simulink model "control_simulation"  (R2016a)
settings: Solver=ode4  StartTime=0.0  StopTime=Tfinal  FixedStep=Ts  RelTol=1e-3
values from neighbouring files (symbols this model uses):
  Cdc = 100e-6    (= 0.0001)    [control_simulation_parameters.m]    (also in pmsm_vbyf_sim_parameters.m = 1.5e-05; vbyfcontrolim_sim.m)
  delta = acos(Ef/Vt)    [control_simulation_parameters.m]    (also in pmsm_vbyf_sim_parameters.m; vbyfcontrolim_sim.m = 0)
  deltad = delta*180/pi    [control_simulation_parameters.m]    (also in pmsm_vbyf_sim_parameters.m)
  Ef = 155    [control_simulation_parameters.m]    (also in pmsm_vbyf_sim_parameters.m = 80)
  fout = 100    [control_simulation_parameters.m]    (also in pmsm_vbyf_sim_parameters.m; vbyfcontrolim_sim.m = 50)
  fsw = 10e3    (= 10000)    [control_simulation_parameters.m]    (also in pmsm_vbyf_sim_parameters.m; vbyfcontrolim_sim.m)
  Ls = 13.8e-3    (= 0.0138)    [control_simulation_parameters.m]
  ma = Vt*sqrt(3)/(Vdcm*0.612)    [control_simulation_parameters.m]    (also in pmsm_vbyf_sim_parameters.m; vbyfcontrolim_sim.m = 0.9)
  motor_speed = 600    [control_simulation_parameters.m]
  phase = [0 90 0 90]    [control_simulation_parameters.m]    (also in pmsm_vbyf_sim_parameters.m = [0])
  Rin = 10    [control_simulation_parameters.m]    (also in pmsm_vbyf_sim_parameters.m = 1; vbyfcontrolim_sim.m = 1e-06)
  Ripth = 0.08    [control_simulation_parameters.m]    (also in pmsm_vbyf_sim_parameters.m; vbyfcontrolim_sim.m)
  Rs = 1e-3    (= 0.001)    [control_simulation_parameters.m]
  Ts = 1e-6    (= 1e-06)    [control_simulation_parameters.m]    (also in pmsm_vbyf_sim_parameters.m; vbyfcontrolim_sim.m)
  Vin = Vdc + Rin*(Pout/Vdc)    (= 697.604412924)    [control_simulation_parameters.m]    (also in pmsm_vbyf_sim_parameters.m = 276.981317008; vbyfcontrolim_sim.m = 750)
  wout = 2*pi*fout    (= 628.318530718)    [control_simulation_parameters.m]    (also in pmsm_vbyf_sim_parameters.m; vbyfcontrolim_sim.m = 314.159265359)
undefined symbols (not defined in the file or in its folder): Lload, Rload
libraries: powerlib x24, powerlib_meascontrol x19, simulink x2
settings Model: Creator=ugurm  LastModifiedBy=mesutto
settings DataIOCC: LimitDataPoints=on  SaveFormat=Array
settings DebuggingCC: UnderspecifiedInitializationDetection=Classic  MergeDetectMultiDrivingBlocksExec=none  SolverPrmCheckMsg=warning  StateNameClashWarn=warning
settings HardwareCC: ProdBitPerPointer=32  ProdLargestAtomicFloat=None  ProdIntDivRoundTo=Undefined  ProdEndianess=Unspecified  ProdWordSize=32  ProdHWDeviceType=32-bit Generic
settings ModelReferenceCC: PropagateSignalLabelsOutOfModel=off
settings ConfigComp: CovModelRefEnable=Off

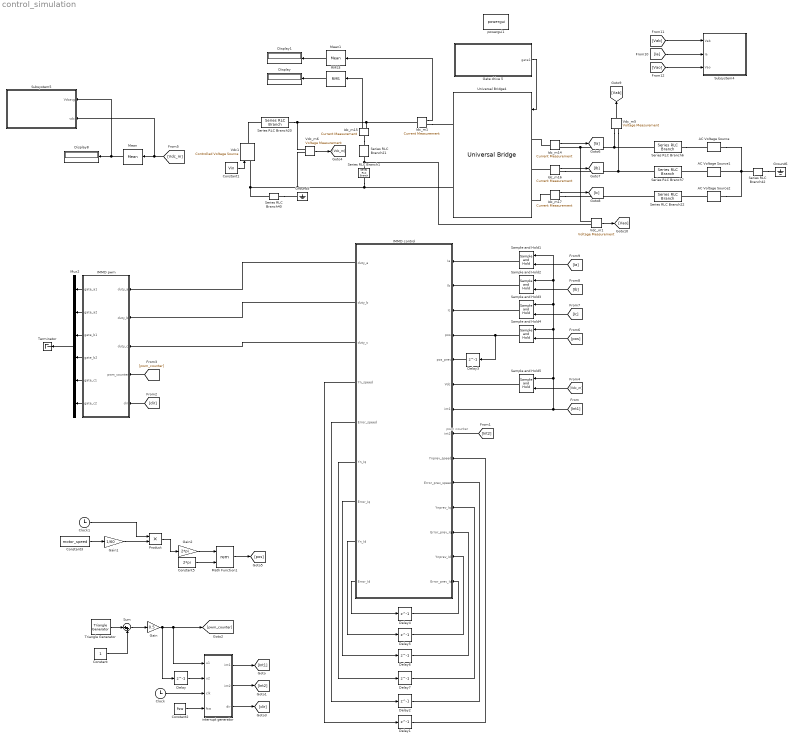
== system control_simulation ==
  note: pwm counter
  AC Voltage Source : powerlib/Electrical Sources/AC Voltage Source  Amplitude=Ef*sqrt(2)  Phase=0  Frequency=fout  SampleTime=0  Measurements=None  BusType=swing  Pref=10e3  Qref=0  Qmin=-inf  Qmax=+inf
  AC Voltage Source1 : powerlib/Electrical Sources/AC Voltage Source  Amplitude=Ef*sqrt(2)  Phase=-120  Frequency=fout  SampleTime=0  Measurements=None  BusType=swing  Pref=10e3  Qref=0  Qmin=-inf  Qmax=+inf
  AC Voltage Source2 : powerlib/Electrical Sources/AC Voltage Source  Amplitude=Ef*sqrt(2)  Phase=-240  Frequency=fout  SampleTime=0  Measurements=None  BusType=swing  Pref=10e3  Qref=0  Qmin=-inf  Qmax=+inf
  Clock : Clock
  Clock1 : Clock
  Constant : Constant
  Constant1 : Constant  Value=Vin
  Constant2 : Constant  Value=fsw
  Constant3 : Constant  Value=motor_speed
  Constant5 : Constant  Value=2*pi
  Delay{,1..7} (8 alike) : Delay  DelayLength=1
  Display : Display
  Display1 : Display
  Display8 : Display
  Gain : Gain  Gain=0.5
  Gain1 : Gain  Gain=1/60
  Gain2 : Gain  Gain=2*pi
  Gate drive 5 : Subsystem
  Ground5 : powerlib/Elements/Ground  LConnTagsString=a
  Ground6 : powerlib/Elements/Ground  LConnTagsString=a
  IMMD control : MATLAB Function  TreatAsAtomicUnit=on
  IMMD pwm : MATLAB Function  TreatAsAtomicUnit=on
  Idc_m{1,14..17} (5 alike) : powerlib/Measurements/Current Measurement  PhasorSimulation=off  OutputType=Complex  PSBequivalent=0
  Math Function1 : Math  Operator=rem  SaturateOnIntegerOverflow=on
  Mean : powerlib_meascontrol/Measurements/Mean  Freq=fout  Vinit=0  Ts=0
  Mean1 : powerlib_meascontrol/Measurements/Mean  Freq=fout  Vinit=0  Ts=0
  Mux2 : Mux  Inputs=6
  Product : Product
  RMS3 : powerlib_meascontrol/Measurements/RMS  TrueRMS=on  Freq=fout  RMSInit=0  Ts=0
  Sample and Hold{1..5} (5 alike) : powerlib_meascontrol/Additional Components/Sample and Hold  ic=0  Ts=0
  Series RLC Branch1 : powerlib/Elements/Series RLC Branch  LConnTagsString=__new0  RConnTagsString=__new0  BranchType=C  Resistance=Rload  Inductance=Lload  SetiL0=off  InitialCurrent=0  Capacitance=Cdc*2  Setx0=off  InitialVoltage=0  Measurements=None
  Series RLC Branch20 : powerlib/Elements/Series RLC Branch  LConnTagsString=__new0  RConnTagsString=__new0  BranchType=R  Resistance=Rin  Inductance=Lload  SetiL0=off  InitialCurrent=0  Capacitance=1e-6  Setx0=off  InitialVoltage=0  Measurements=None
  Series RLC Branch21 : powerlib/Elements/Series RLC Branch  LConnTagsString=__new0  RConnTagsString=__new0  BranchType=C  Resistance=Rload  Inductance=Lload  SetiL0=off  InitialCurrent=0  Capacitance=Cdc*2  Setx0=off  InitialVoltage=0  Measurements=None
  Series RLC Branch22 : powerlib/Elements/Series RLC Branch  LConnTagsString=__new0  RConnTagsString=__new0  BranchType=RL  Resistance=Rs  Inductance=Ls  SetiL0=off  InitialCurrent=0  Capacitance=1e-6  Setx0=off  InitialVoltage=0  Measurements=None
  Series RLC Branch40 : powerlib/Elements/Series RLC Branch  LConnTagsString=__new0  RConnTagsString=__new0  BranchType=R  Resistance=1e12  Inductance=Lload  SetiL0=off  InitialCurrent=0  Capacitance=1e-6  Setx0=off  InitialVoltage=0  Measurements=None
  Series RLC Branch42 : powerlib/Elements/Series RLC Branch  LConnTagsString=__new0  RConnTagsString=__new0  BranchType=R  Resistance=1e12  Inductance=Lload  SetiL0=off  InitialCurrent=0  Capacitance=1e-6  Setx0=off  InitialVoltage=0  Measurements=None
  Series RLC Branch6 : powerlib/Elements/Series RLC Branch  LConnTagsString=__new0  RConnTagsString=__new0  BranchType=RL  Resistance=Rs  Inductance=Ls  SetiL0=off  InitialCurrent=0  Capacitance=1e-6  Setx0=off  InitialVoltage=0  Measurements=None
  Series RLC Branch7 : powerlib/Elements/Series RLC Branch  LConnTagsString=__new0  RConnTagsString=__new0  BranchType=RL  Resistance=Rs  Inductance=Ls  SetiL0=off  InitialCurrent=0  Capacitance=1e-6  Setx0=off  InitialVoltage=0  Measurements=None
  Subsystem4 : Subsystem
  Subsystem5 : Subsystem
  Sum : Sum  Inputs=|++
  Terminator : Terminator
  Triangle Generator : powerlib_meascontrol/Pulse & Signal Generators/Triangle Generator  Freq=fsw  Phase=0  Ts=0
  Universal Bridge4 : powerlib/Power Electronics/Universal Bridge  Arms=3  SnubberResistance=1e5  SnubberCapacitance=inf  Device=IGBT / Diodes  Ron=1e-6  Lon=0  ForwardVoltages="[  0  0  ]"  ForwardVoltage=0  GTOparameters=[ 10e-6 , 20e-6 ]  IGBTparameters=[0,0]  Measurements=None  Measurements_2=None  converterType=Rectifier
  Vdc1 : powerlib/Electrical Sources/Controlled Voltage Source  Initialize=off  Source_Type=DC  Amplitude=200  Phase=0  Frequency=0  Measurements=None
  Vdc_m1 : powerlib/Measurements/Voltage Measurement  PhasorSimulation=off  OutputType=Complex  PSBequivalent=0
  Vdc_m5 : powerlib/Measurements/Voltage Measurement  PhasorSimulation=off  OutputType=Complex  PSBequivalent=0
  Vdc_m6 : powerlib/Measurements/Voltage Measurement  PhasorSimulation=off  OutputType=Complex  PSBequivalent=0
  interrupt generator : MATLAB Function  TreatAsAtomicUnit=on
  powergui1 : powerlib/powergui  Priority=1  SimulationMode=Discrete  SolverType=Tustin  SampleTime=Ts  frequency=60  SPID=off  DisableSnubberDevices=off  DisableRonSwitches=off  DisableVfSwitches=off  SwTol=0  DisplayEquations=off  Interpol=off  ExternalGateDelay=off  methode=off  Ts=0  FunctionMessages=off  echomessages=off  HookPort=off  EnableUseOfTLC=off  x0status=blocks  frequencyindice=0  Pbase=100e6  ErrMax=1e-4  Iterations=50  UnitsV=kV  UnitsW=MW  buscounter=0  RestoreLinks=warning  ResistiveCurrentMeasurement=off  Frange=[0:2:500]  Ylog=off  Xlog=on  ShowGrid=off  save=off  variable=ZData  structure=Vdc  ZoomFFT=off  StartTime=0.04  cycles=5  DisplayStyle=5  fundamental=50  FreqAxis=off  MaxFrequency=30000  frequencyindicesteady=1  RmsSteady=1  display=off
  wires:
  Gate drive 5/1(gate1) -> Universal Bridge4/1
  Constant1/1 -> Vdc1/1
  Idc_m15/1 -> RMS3/1
  Vdc_m6/1 -> [Vdc_m]
  RMS3/1 -> Display/1
  Mean/1 -> Subsystem5/1(Vdcavg), Display8/1
  Idc_m1/1 -> Mean1/1
  Mean1/1 -> Display1/1
  Triangle Generator/1 -> Sum/1
  Constant/1 -> Sum/2
  Sum/1 -> Gain/1
  Gain/1 -> [pwm_counter], interrupt generator/1(u1), Delay/1
  Delay/1 -> interrupt generator/2(u2)
  Clock/1 -> interrupt generator/3(clk)
  Constant2/1 -> interrupt generator/4(fsw)
  Idc_m14/1 -> [Ia]
  [Int1] -> IMMD control/7(int1), Sample and Hold4/2, Sample and Hold3/2, Sample and Hold2/2, Sample and Hold1/2, Sample and Hold5/2
  Constant3/1 -> Gain1/1
  Gain1/1 -> Product/2
  Clock1/1 -> Product/1
  Product/1 -> Gain2/1
  Gain2/1 -> Math Function1/1
  Constant5/1 -> Math Function1/2
  IMMD pwm/1(gate_a1) -> Mux2/1
  IMMD pwm/2(gate_a2) -> Mux2/2
  IMMD pwm/3(gate_b1) -> Mux2/3
  IMMD pwm/4(gate_b2) -> Mux2/4
  IMMD pwm/5(gate_c1) -> Mux2/5
  IMMD pwm/6(gate_c2) -> Mux2/6
  Sample and Hold4/1 -> Delay3/1, IMMD control/4(pos)
  Sample and Hold3/1 -> IMMD control/3(Ic)
  Sample and Hold2/1 -> IMMD control/2(Ib)
  Sample and Hold1/1 -> IMMD control/1(Ia)
  Sample and Hold5/1 -> IMMD control/6(Vdc)
  IMMD control/4(Yn_speed) -> Delay1/1
  Delay1/1 -> IMMD control/9(Ynprev_speed)
  IMMD control/5(Error_speed) -> Delay2/1
  Delay2/1 -> IMMD control/10(Error_prev_speed)
  interrupt generator/1(int1) -> [Int1]
  Mux2/1 -> Terminator/1
  Delay3/1 -> IMMD control/5(pos_prev)
  interrupt generator/2(int2) -> [Int2]
  [Int2] -> IMMD control/8(int2)
  [dir] -> IMMD pwm/5(dir)
  interrupt generator/3(dir) -> [dir]
  [pwm_counter] -> IMMD pwm/4(pwm_counter)
  [Vdc_m] -> Sample and Hold5/1
  IMMD control/9(Error_Id) -> Delay4/1
  Delay4/1 -> IMMD control/14(Error_prev_Id)
  Delay5/1 -> IMMD control/13(Ynprev_Id)
  Delay6/1 -> IMMD control/12(Error_prev_Iq)
  Delay7/1 -> IMMD control/11(Ynprev_Iq)
  IMMD control/6(Yn_Iq) -> Delay7/1
  IMMD control/8(Yn_Id) -> Delay5/1
  IMMD control/7(Error_Iq) -> Delay6/1
  IMMD control/3(duty_c) -> IMMD pwm/3(duty_c)
  IMMD control/2(duty_b) -> IMMD pwm/2(duty_b)
  IMMD control/1(duty_a) -> IMMD pwm/1(duty_a)
  [Vdc_m] -> Subsystem5/2(vdc), Mean/1
  [pos] -> Sample and Hold4/1
  Math Function1/1 -> [pos]
  [Ia] -> Sample and Hold1/1
  [Ib] -> Sample and Hold2/1
  [Ic] -> Sample and Hold3/1
  [Ia] -> Subsystem4/2(Ia)
  Idc_m16/1 -> [Ib]
  Idc_m17/1 -> [Ic]
  [Vab] -> Subsystem4/1(Vab)
  [Vao] -> Subsystem4/3(Vao)
  Vdc_m5/1 -> [Vab]
  Vdc_m1/1 -> [Vao]
  connections:
  Vdc_m5/LConn1 -- Idc_m14/RConn1 -- Vdc_m1/LConn1 -- Series RLC Branch6/LConn1
  Universal Bridge4/RConn2 -- Vdc_m6/LConn2 -- Vdc1/LConn1 -- Series RLC Branch40/LConn1 -- Series RLC Branch1/RConn1
  Series RLC Branch42/RConn1 -- Ground6/LConn1
  Series RLC Branch40/RConn1 -- Ground5/LConn1
  Idc_m14/LConn1 -- Universal Bridge4/LConn1
  Idc_m15/LConn1 -- Series RLC Branch21/LConn1
  Vdc1/RConn1 -- Series RLC Branch20/LConn1
  Series RLC Branch6/RConn1 -- AC Voltage Source/RConn1
  AC Voltage Source1/RConn1 -- Series RLC Branch7/RConn1
  AC Voltage Source2/RConn1 -- Series RLC Branch22/RConn1
  Series RLC Branch42/LConn1 -- AC Voltage Source/LConn1 -- AC Voltage Source2/LConn1 -- AC Voltage Source1/LConn1
  Idc_m16/LConn1 -- Universal Bridge4/LConn2
  Idc_m17/LConn1 -- Universal Bridge4/LConn3
  Idc_m17/RConn1 -- Series RLC Branch22/LConn1
  Idc_m16/RConn1 -- Vdc_m5/LConn2 -- Series RLC Branch7/LConn1
  Idc_m1/RConn1 -- Universal Bridge4/RConn1
  Idc_m1/LConn1 -- Series RLC Branch20/RConn1 -- Vdc_m6/LConn1 -- Idc_m15/RConn1
  Series RLC Branch1/LConn1 -- Vdc_m1/LConn2 -- Series RLC Branch21/RConn1

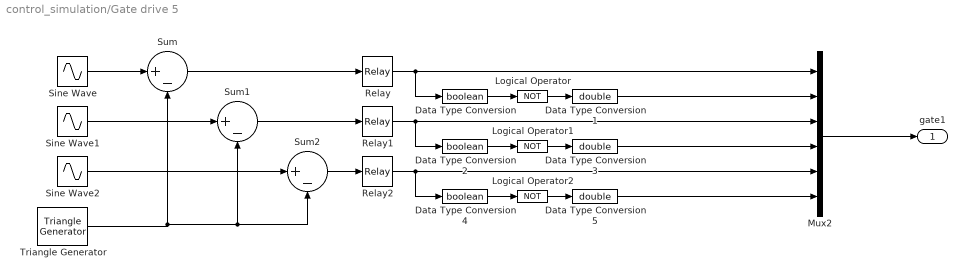
== system control_simulation/Gate drive 5 ==
  Data Type Conversion : DataTypeConversion  OutDataTypeStr=boolean
  Data Type Conversion1 : DataTypeConversion  OutDataTypeStr=double
  Data Type Conversion2 : DataTypeConversion  OutDataTypeStr=boolean
  Data Type Conversion3 : DataTypeConversion  OutDataTypeStr=double
  Data Type Conversion4 : DataTypeConversion  OutDataTypeStr=boolean
  Data Type Conversion5 : DataTypeConversion  OutDataTypeStr=double
  Logical Operator : Logic  Operator=NOT  AllPortsSameDT=off  OutDataTypeStr=boolean
  Logical Operator1 : Logic  Operator=NOT  AllPortsSameDT=off  OutDataTypeStr=boolean
  Logical Operator2 : Logic  Operator=NOT  AllPortsSameDT=off  OutDataTypeStr=boolean
  Mux2 : Mux  Inputs=6
  Relay : Relay
  Relay1 : Relay
  Relay2 : Relay
  Sine Wave : Sin  Amplitude=ma  Frequency=wout  Phase=delta  SampleTime=0
  Sine Wave1 : Sin  Amplitude=ma  Frequency=wout  Phase=-2*pi/3+delta  SampleTime=0
  Sine Wave2 : Sin  Amplitude=ma  Frequency=wout  Phase=2*pi/3+delta  SampleTime=0
  Sum : Sum  Inputs=|+-
  Sum1 : Sum  Inputs=|+-
  Sum2 : Sum  Inputs=|+-
  Triangle Generator : powerlib_meascontrol/Pulse & Signal Generators/Triangle Generator  Freq=fsw  Phase=phase(1)  Ts=Ts
  gate1 : Outport
  wires:
  Sine Wave/1 -> Sum/1
  Triangle Generator/1 -> Sum1/2, Sum2/2, Sum/2
  Sine Wave1/1 -> Sum1/1
  Sine Wave2/1 -> Sum2/1
  Sum/1 -> Relay/1
  Sum1/1 -> Relay1/1
  Sum2/1 -> Relay2/1
  Data Type Conversion/1 -> Logical Operator/1
  Relay/1 -> Data Type Conversion/1, Mux2/1
  Logical Operator/1 -> Data Type Conversion1/1
  Data Type Conversion1/1 -> Mux2/2
  Data Type Conversion2/1 -> Logical Operator1/1
  Relay1/1 -> Data Type Conversion2/1, Mux2/3
  Logical Operator1/1 -> Data Type Conversion3/1
  Data Type Conversion3/1 -> Mux2/4
  Data Type Conversion4/1 -> Logical Operator2/1
  Relay2/1 -> Data Type Conversion4/1, Mux2/5
  Logical Operator2/1 -> Data Type Conversion5/1
  Data Type Conversion5/1 -> Mux2/6
  Mux2/1 -> gate1/1

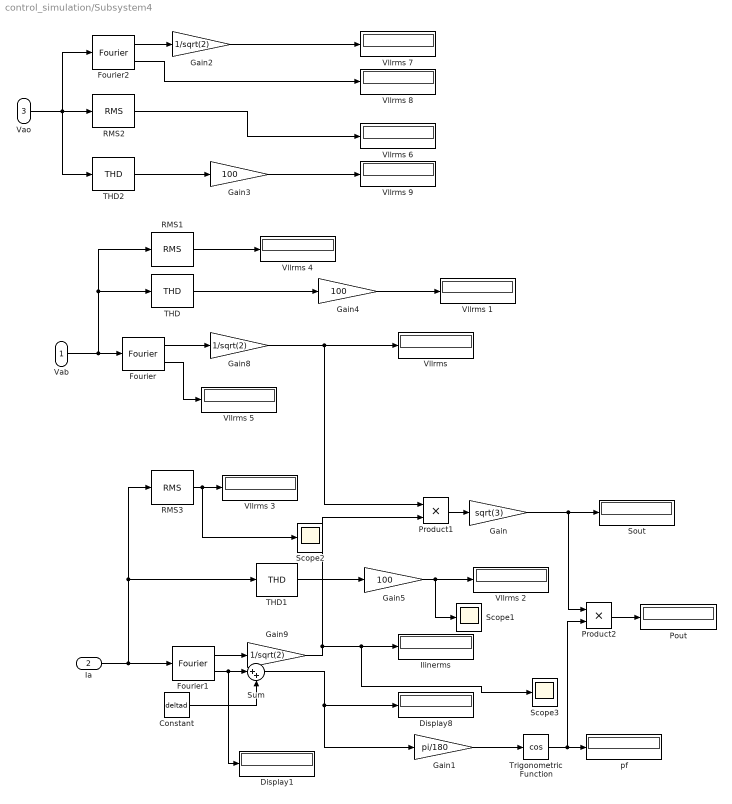
== system control_simulation/Subsystem4 ==
  Vab : Inport
  Ia : Inport  Port=2
  Vao : Inport  Port=3
  Constant : Constant  Value=deltad
  Display1 : Display
  Display8 : Display
  Fourier : powerlib_meascontrol/Measurements/Fourier  Freq=fout  n=1  InInit=[0, 0]  Ts=Ts
  Fourier1 : powerlib_meascontrol/Measurements/Fourier  Freq=fout  n=1  InInit=[0, 0]  Ts=Ts
  Fourier2 : powerlib_meascontrol/Measurements/Fourier  Freq=fout  n=1  InInit=[0, 0]  Ts=Ts
  Gain : Gain  Gain=sqrt(3)
  Gain1 : Gain  Gain=pi/180
  Gain2 : Gain  Gain=1/sqrt(2)
  Gain3 : Gain  Gain=100
  Gain4 : Gain  Gain=100
  Gain5 : Gain  Gain=100
  Gain8 : Gain  Gain=1/sqrt(2)
  Gain9 : Gain  Gain=1/sqrt(2)
  "Ilinerms " : Display
  Pout : Display
  Product1 : Product
  Product2 : Product
  RMS1 : powerlib_meascontrol/Measurements/RMS  TrueRMS=on  Freq=fout  RMSInit=0  Ts=0
  RMS2 : powerlib_meascontrol/Measurements/RMS  TrueRMS=on  Freq=fout  RMSInit=0  Ts=0
  RMS3 : powerlib_meascontrol/Measurements/RMS  TrueRMS=on  Freq=fout  RMSInit=0  Ts=0
  Scope1 : Scope
  Scope2 : Scope
  Scope3 : Scope
  Sout : Display
      settings: Format=short_e
  Sum : Sum  Inputs=|++
  THD : powerlib_meascontrol/Measurements/THD  Freq=fout  Ts=0
  THD1 : powerlib_meascontrol/Measurements/THD  Freq=fout  Ts=0
  THD2 : powerlib_meascontrol/Measurements/THD  Freq=fout  Ts=0
  Trigonometric Function : Trigonometry  Operator=cos
  Vllrms {,1..9} (10 alike) : Display
  pf : Display
  wires:
  Gain8/1 -> Product1/1, "Vllrms "/1
  Gain9/1 -> Scope3/1, "Ilinerms "/1, Product1/2
  Ia/1 -> RMS3/1, THD1/1, Fourier1/1
  Fourier1/1 -> Gain9/1
  Vab/1 -> RMS1/1, THD/1, Fourier/1
  Fourier/1 -> Gain8/1
  Product1/1 -> Gain/1
  Gain/1 -> Product2/1, Sout/1
  Sum/1 -> Gain1/1, Display8/1
  Trigonometric Function/1 -> Product2/2, pf/1
  Gain1/1 -> Trigonometric Function/1
  Product2/1 -> Pout/1
  Fourier/2 -> Vllrms 5/1
  THD/1 -> Gain4/1
  THD1/1 -> Gain5/1
  Constant/1 -> Sum/2
  RMS3/1 -> Scope2/1, Vllrms 3/1
  RMS1/1 -> Vllrms 4/1
  Fourier1/2 -> Display1/1, Sum/1
  Vao/1 -> THD2/1, Fourier2/1, RMS2/1
  RMS2/1 -> Vllrms 6/1
  Fourier2/1 -> Gain2/1
  Fourier2/2 -> Vllrms 8/1
  Gain2/1 -> Vllrms 7/1
  THD2/1 -> Gain3/1
  Gain3/1 -> Vllrms 9/1
  Gain4/1 -> Vllrms 1/1
  Gain5/1 -> Scope1/1, Vllrms 2/1

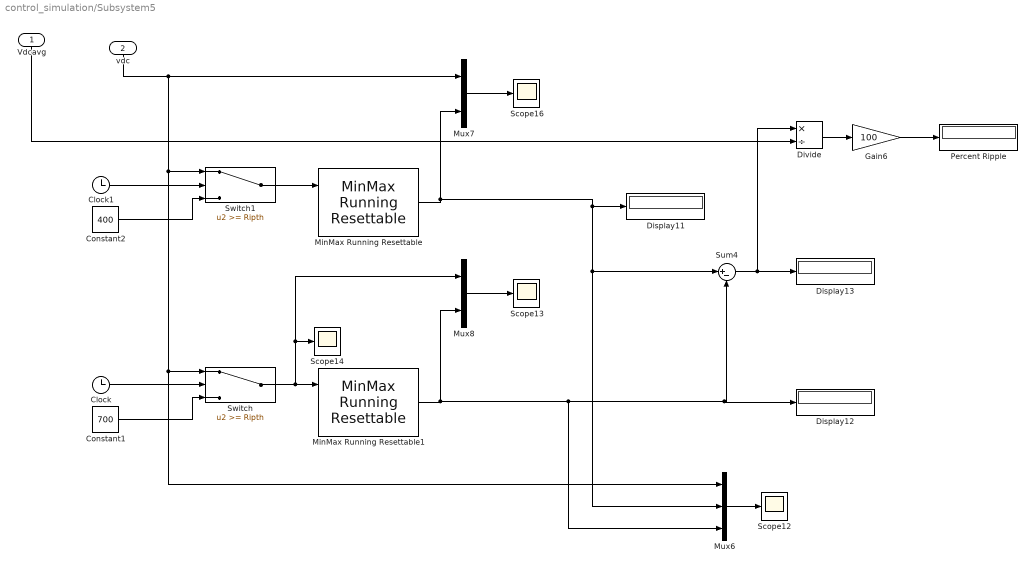
== system control_simulation/Subsystem5 ==
  Vdcavg : Inport
  vdc : Inport  Port=2
  Clock : Clock
  Clock1 : Clock
  Constant1 : Constant  Value=700  SampleTime=Ts
  Constant2 : Constant  Value=400  SampleTime=Ts
  Display11 : Display
  Display12 : Display
  Display13 : Display
  Divide : Product  Inputs=*/
  Gain6 : Gain  Gain=100
  MinMax Running Resettable : simulink/Math Operations/MinMax Running Resettable  Function=max  vinit=0.0
  MinMax Running Resettable1 : simulink/Math Operations/MinMax Running Resettable  Function=min  vinit=700
  Mux6 : Mux  Inputs=3
  Mux7 : Mux  Inputs=2
  Mux8 : Mux  Inputs=2
  Percent Ripple : Display
  Scope{12..14,16} (4 alike) : Scope
  Sum4 : Sum  Inputs=|+-
  Switch : Switch  Threshold=Ripth
  Switch1 : Switch  Threshold=Ripth
  wires:
  MinMax Running Resettable/1 -> Display11/1, Mux6/2, Sum4/1, Mux7/2
  Clock/1 -> Switch/2
  Mux8/1 -> Scope13/1
  Gain6/1 -> Percent Ripple/1
  Constant1/1 -> Switch/3
  MinMax Running Resettable1/1 -> Mux6/3, Display12/1, Sum4/2, Mux8/2
  Mux7/1 -> Scope16/1
  Switch/1 -> Mux8/1, Scope14/1, MinMax Running Resettable1/1
  Sum4/1 -> Divide/1, Display13/1
  Divide/1 -> Gain6/1
  Mux6/1 -> Scope12/1
  Vdcavg/1 -> Divide/2
  vdc/1 -> Mux7/1, Switch1/1, Mux6/1, Switch/1
  Switch1/1 -> MinMax Running Resettable/1
  Clock1/1 -> Switch1/2
  Constant2/1 -> Switch1/3

== matlab function control_simulation/IMMD control ==
  data: Ia input; duty_a output; Ib input; Ic input; pos input; pos_prev input; Vdc input; duty_b output; duty_c output; int1 input; int2 input; Ynprev_speed input; Error_prev_speed input; Yn_speed output; Error_speed output; Ynprev_Iq input; Error_prev_Iq input; Ynprev_Id input; Error_prev_Id input; Yn_Iq output; Error_Iq output; Yn_Id output; Error_Id output
function [duty_a,duty_b,duty_c,Yn_speed,Error_speed,...
          Yn_Iq,Error_Iq,Yn_Id,Error_Id] = fcn(...
    Ia,Ib,Ic,pos,pos_prev,Vdc,int1,int2,...
    Ynprev_speed,Error_prev_speed,...
    Ynprev_Iq,Error_prev_Iq,Ynprev_Id,Error_prev_Id)

pole_pair = 10;
fsw = 10000; % Hz
Vdc_ref = 540; % V

if (int1 == 1) % interrupt on zero event

    % DC link voltage average
    
    
    % DC link voltage control
    
    
    % Speed from position
    delta_T = 1/fsw;
    Speed = (pos - pos_prev)/delta_T; % rad/sec
    Pos_Elec = pos*pole_pair; % rad
    
    % PI for speed
    Kp_speed = 10;
    Ki_speed = 5;
    Ymax_speed = 100;
    Ymin_speed = -100;
    Speed_ref = 600; % rpm
    Error_speed = Speed_ref - Speed;
    Yn_speed = Ynprev_speed + Error_speed*(Kp_speed+Ki_speed)...
        - Error_prev_speed*(Kp_speed);
    if (Yn_speed > Ymax_speed)
        Yn_speed = Ymax_speed;
    elseif (Yn_speed < Ymin_speed)
        Yn_speed = Ymin_speed;
    end
    
    % clarke transform for currents
    Ialfa = (2/3)*Ia - (1/3)*(Ib + Ic);
    Ibeta = (1/sqrt(3))*(Ib - Ic);
    
    % park transform for currents
    Id = Ialfa*cos(Pos_Elec) + Ibeta*sin(Pos_Elec);   
    Iq = Ialfa*sin(Pos_Elec) - Ibeta*cos(Pos_Elec);   
    
    % iq control
    Kp_Iq = 10;
    Ki_Iq = 5;
    Ymax_Iq = 100;
    Ymin_Iq = -100;
    Iq_ref = 0;
    Error_Iq = Iq_ref - Iq;
    Yn_Iq = Ynprev_Iq + Error_Iq*(Kp_Iq+Ki_Iq)...
        - Error_prev_Iq*(Kp_Iq);     
    if (Yn_Iq > Ymax_Iq)
        Yn_Iq = Ymax_Iq;
    elseif (Yn_Iq < Ymin_Iq)
        Yn_Iq = Ymin_Iq;
    end
    
    % id control
    Kp_Id = 10;
    Ki_Id = 5;
    Ymax_Id = 100;
    Ymin_Id = -100;
    Id_ref = Yn_speed; 
    Error_Id = Id_ref - Id;
    Yn_Id = Ynprev_Id + Error_Id*(Kp_Id+Ki_Id)...
        - Error_prev_Id*(Kp_Id);  
    if (Yn_Id > Ymax_Id)
        Yn_Id = Ymax_Id;
    elseif (Yn_Id < Ymin_Id)
        Yn_Id = Ymin_Id;
    end
    
    % Assign voltage references
    Vd = Yn_Id;
    Vq = Yn_Iq;
    
    % inverse park transform for currents
    Valfa = Vd*cos(Pos_Elec) + Vq*sin(Pos_Elec);   
    Vbeta = -Vq*cos(Pos_Elec) + Vd*sin(Pos_Elec);   
    
    % inverse clarke transform for currents
    Va_ref = Valfa;
    Vb_ref = (-Valfa + sqrt(3)*Vbeta)/2;
    Vc_ref = (-Valfa - sqrt(3)*Vbeta)/2;
        
    duty_a_temp = Va_ref/Vdc_ref;
    duty_b_temp = Vb_ref/Vdc_ref;
    duty_c_temp = Vc_ref/Vdc_ref;
    
else
    duty_a_temp = 1; %//
    duty_b_temp = 1; %//
    duty_c_temp = 1; %//
    Yn_speed = Ynprev_speed;
    Error_speed = Error_prev_speed;
    Yn_Iq = Ynprev_Iq;
    Error_Iq = Error_prev_Iq;    
    Yn_Id = Ynprev_Id;
    Error_Id = Error_prev_Id;
end;

if (int2 == 1) % interrupt on prd event
    duty_a = duty_a_temp;
    duty_b = duty_b_temp;
    duty_c = duty_c_temp;
else
    duty_a = 1; %//
    duty_b = 1; %//
    duty_c = 1; %//
end;

== matlab function control_simulation/interrupt generator ==
  data: u1 input; int1 output; u2 input; clk input; int2 output; dir output; fsw input
function [int1,int2,dir] = fcn(u1,u2,clk,fsw)

if (rem(clk,1/fsw) == 0)
    int1 = 1; % interrupt on zero
    dir = 0;
else
    int1 = 0;
    if (u1 > u2)
        dir = 1; % up
    else
        dir = 0; % down
    end;
end;

if (rem(clk*2,1/fsw) == 0 && rem(clk,1/fsw) ~= 0)
    int2 = 1; % interrupt on period
else
    int2 = 0;
end;

== matlab function control_simulation/IMMD pwm ==
  data: duty_a input; gate_a1 output; duty_b input; duty_c input; gate_a2 output; gate_b1 output; gate_b2 output; gate_c1 output; gate_c2 output; pwm_counter input; dir input
function [gate_a1,gate_a2,gate_b1,gate_b2,gate_c1,gate_c2] = fcn(duty_a,duty_b,duty_c,pwm_counter,dir)

%if (dir == 1)
    if (duty_a > pwm_counter)
        gate_a1 = 1;
        gate_a2 = 0;
    else
        gate_a1 = 0;
        gate_a2 = 1;
    end;
    if (duty_b > pwm_counter)
        gate_b1 = 1;
        gate_b2 = 0;
    else
        gate_b1 = 0;
        gate_b2 = 1;
    end;
    if (duty_c > pwm_counter)
        gate_c1 = 1;
        gate_c2 = 0;
    else
        gate_c1 = 0;
        gate_c2 = 1;
    end;

%else
    

%end;
